simulink model "P1_DiegoGonzalezAtziriDaniela"  (R2023b)
settings: Solver=ode23  StartTime=0.0  StopTime=200  RelTol=1e-3
settings Model: Creator=danid  LastModifiedBy=danid

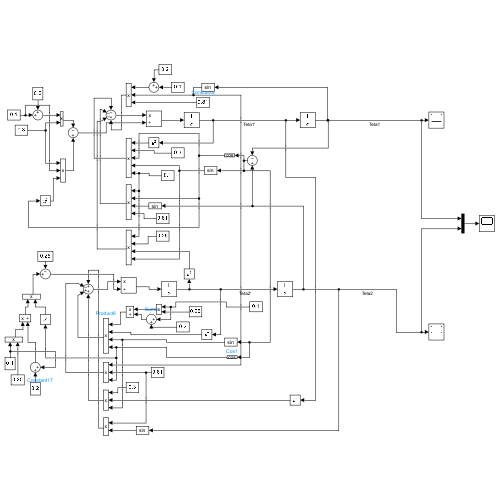
[thumbnail: Simulink's stored preview of the top-level diagram]
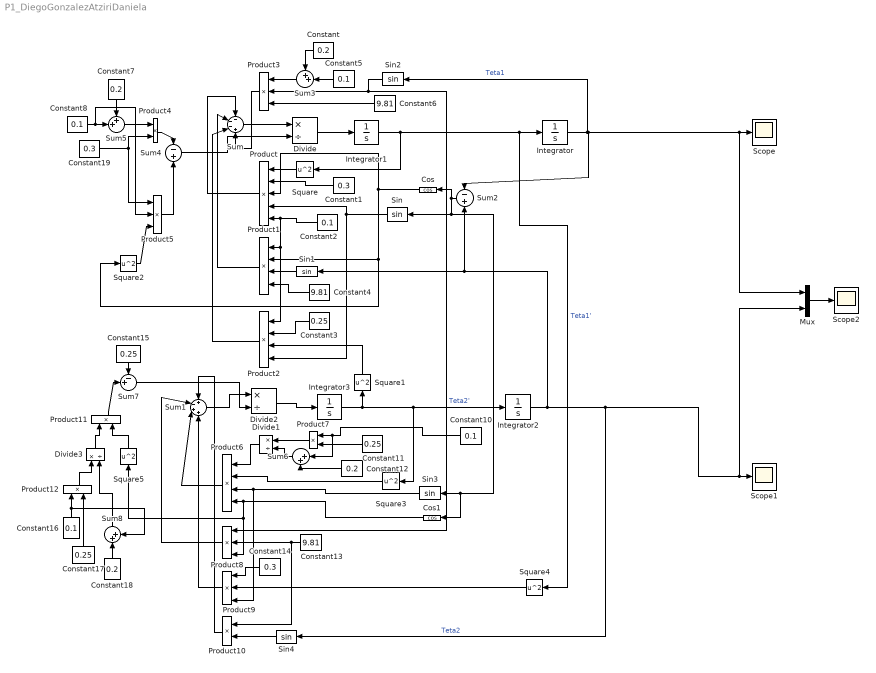
== system P1_DiegoGonzalezAtziriDaniela ==
  Constant{,7,12,18} (4 alike) : Constant  Value=0.2
  Constant1 : Constant  Value=0.3
  Constant{2,5,8,10,16} (5 alike) : Constant  Value=0.1
  Constant{3,11,15,17} (4 alike) : Constant  Value=0.25
  Constant13 : Constant  Value=9.81
  Constant14 : Constant  Value=0.3
  Constant19 : Constant  Value=0.3
  Constant4 : Constant  Value=9.81
  Constant6 : Constant  Value=9.81
  Cos : Trigonometry  Operator=cos
  Cos1 : Trigonometry  Operator=cos
  Divide{,1..3} (4 alike) : Product  Inputs=*/
  Integrator : Integrator
  Integrator1 : Integrator
  Integrator2 : Integrator  InitialCondition=0.610865
  Integrator3 : Integrator
  Mux : Mux  Inputs=2
  Product : Product  Inputs=5
  Product1 : Product  Inputs=4
  Product{4,7,10..12} (5 alike) : Product
  Product2 : Product  Inputs=4
  Product{3,5,8..9} (4 alike) : Product  Inputs=3
  Product6 : Product  Inputs=4
  Scope : Scope
  Scope1 : Scope
  Scope2 : Scope
  Sin{,1..4} (5 alike) : Trigonometry
  Square{,1..5} (6 alike) : Math  Operator=square
  Sum : Sum  Inputs=---+
  Sum1 : Sum  Inputs=+-++
  Sum2 : Sum  Inputs=-+
  Sum3 : Sum  Inputs=++|
  Sum4 : Sum  Inputs=-+
  Sum5 : Sum  Inputs=++|
  Sum6 : Sum  Inputs=|++
  Sum7 : Sum  Inputs=-+|
  Sum8 : Sum  Inputs=|++
  wires:
  Integrator1/1 -> Square/1, Square4/1, Integrator/1  "Teta1'"
  Integrator/1 -> Sin2/1, Sum2/1, Mux/1, Scope/1  "Teta1"
  Integrator3/1 -> Square1/1, Square3/1, Integrator2/1  "Teta2'"
  Integrator2/1 -> Sum2/2, Sin1/1, Sin4/1, Mux/2, Scope1/1  "Teta2"
  Divide/1 -> Integrator1/1
  Sum/1 -> Divide/1
  Product/1 -> Sum/1
  Square/1 -> Product/1
  Constant1/1 -> Product/2
  Constant2/1 -> Product2/1, Product1/1, Product/5
  Sin/1 -> Product2/4, Product/4
  Cos/1 -> Product1/2, Square2/1, Product/3
  Sum2/1 -> Cos1/1, Sin3/1, Sin/1, Cos/1
  Product1/1 -> Sum/2
  Constant4/1 -> Product1/4
  Sin1/1 -> Product1/3
  Product2/1 -> Sum/3
  Constant3/1 -> Product2/2
  Square1/1 -> Product2/3
  Product3/1 -> Sum/4
  Sum3/1 -> Product3/1
  Constant/1 -> Sum3/1
  Constant5/1 -> Sum3/2
  Constant6/1 -> Product3/3
  Sin2/1 -> Product8/1, Product3/2
  Sum5/1 -> Product4/1
  Product4/1 -> Sum4/1
  Constant7/1 -> Sum5/1
  Constant8/1 -> Product5/2, Sum5/2
  Constant19/1 -> Product5/1, Product4/2
  Sum4/1 -> Divide/2
  Product5/1 -> Sum4/2
  Square2/1 -> Product5/3
  Divide1/1 -> Product6/1
  Constant11/1 -> Product7/2
  Constant10/1 -> Sum6/1, Product7/1
  Product7/1 -> Divide1/1
  Sum6/1 -> Divide1/2
  Constant12/1 -> Sum6/2
  Square3/1 -> Product6/2
  Sin3/1 -> Product6/3, Product9/3
  Cos1/1 -> Product8/3, Square5/1, Product6/4
  Product6/1 -> Sum1/3
  Constant13/1 -> Product10/1, Product8/2
  Product8/1 -> Sum1/2
  Product9/1 -> Sum1/4
  Divide2/1 -> Integrator3/1
  Constant14/1 -> Product9/1
  Square4/1 -> Product9/2
  Sin4/1 -> Product10/2
  Constant15/1 -> Sum7/1
  Product11/1 -> Sum7/2
  Square5/1 -> Product11/2
  Divide3/1 -> Product11/1
  Product12/1 -> Divide3/1
  Constant16/1 -> Sum8/2, Product12/1
  Constant17/1 -> Product12/2
  Sum8/1 -> Divide3/2
  Constant18/1 -> Sum8/1
  Mux/1 -> Scope2/1
  Sum1/1 -> Divide2/1
  Sum7/1 -> Divide2/2
  Product10/1 -> Sum1/1
